simulink model "simulation32"  (R2015b)
settings: Solver=VariableStepAuto  StartTime=0.0  StopTime=1500  RelTol=1e-3
values from neighbouring files (symbols this model uses):
  A = [ ... (first row only)    [stateSpaceModel.m]
  B = [ ... (first row only)    [stateSpaceModel.m]
  C = [ ... (first row only)    [stateSpaceModel.m]
  C_2 = [ ... (first row only)    [stateSpaceModel.m]
  D = [ ... (first row only)    [stateSpaceModel.m]
  D_2 = [ ... (first row only)    [stateSpaceModel.m]
  g = 9.81    [constantsForControlGains.m]
  step_course_hold = 25    [stepsForCourseHoldAndManeuvers.m]
  step_course_hold_start_time = 200    [stepsForCourseHoldAndManeuvers.m]
  step_manuever1 = 20    [stepsForCourseHoldAndManeuvers.m]
  step_manuever1_start_time = 200    [stepsForCourseHoldAndManeuvers.m]
  step_manuever2 = 60    [stepsForCourseHoldAndManeuvers.m]
  step_manuever2_start_time = 400    [stepsForCourseHoldAndManeuvers.m]
  step_manuever3 = 70    [stepsForCourseHoldAndManeuvers.m]
  step_manuever3_start_time = 600    [stepsForCourseHoldAndManeuvers.m]
  step_manuever4 = -50    [stepsForCourseHoldAndManeuvers.m]
  step_manuever4_start_time = 800    [stepsForCourseHoldAndManeuvers.m]
  step_manuever5 = -80    [stepsForCourseHoldAndManeuvers.m]
  step_manuever5_start_time = 1000    [stepsForCourseHoldAndManeuvers.m]
  step_manuever6 = -60    [stepsForCourseHoldAndManeuvers.m]
  step_manuever6_start_time = 1200    [stepsForCourseHoldAndManeuvers.m]
  T = 20    [stepsForCourseHoldAndManeuvers.m]
  Va = 552/3.6    (= 153.333333333)    [constantsForControlGains.m]
undefined symbols (not defined in the file or in its folder): Kp, Kphi, Kr, T_chi, Tw
libraries: simulink_extras x11
settings Model: Creator=ShivJeet  LastModifiedBy=ShivJeet

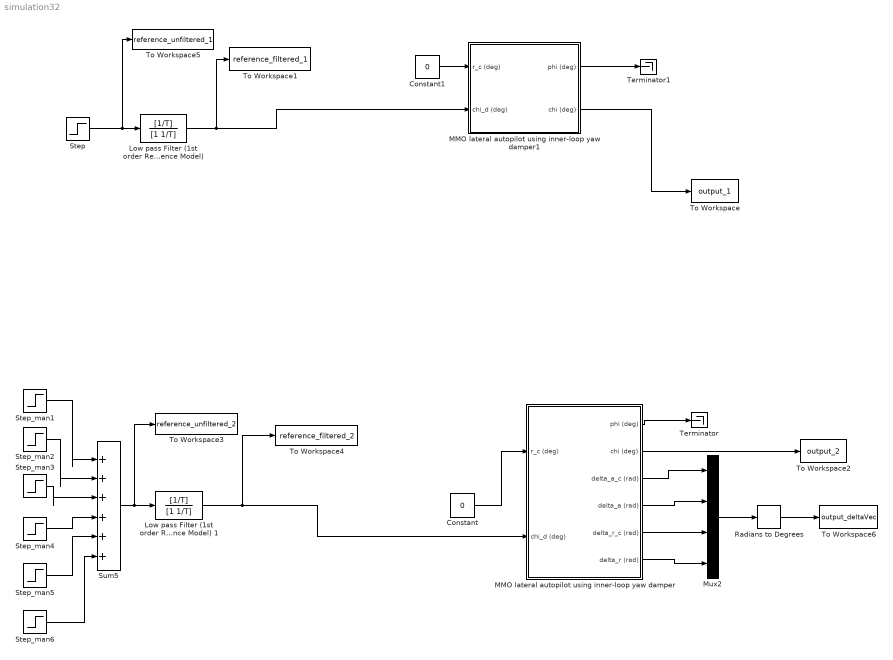
== system simulation32 ==
  Constant : Constant  Value=0
  Constant1 : Constant  Value=0
  "Low pass Filter (1st order Reference Model) " : TransferFcn  Numerator=[1/T]  Denominator=[1 1/T]
  Low pass Filter (1st order Reference Model) 1 : TransferFcn  Numerator=[1/T]  Denominator=[1 1/T]
  MMO lateral autopilot using inner-loop yaw damper : Subsystem
  MMO lateral autopilot using inner-loop yaw damper1 : Subsystem
  Mux2 : Mux
  Radians to Degrees : simulink_extras/Transformations/Radians to Degrees
  Step : Step  Time=step_course_hold_start_time  After=step_course_hold  SampleTime=0
  Step_man1 : Step  Time=step_manuever1_start_time  After=step_manuever1  SampleTime=0
  Step_man2 : Step  Time=step_manuever2_start_time  After=step_manuever2  SampleTime=0
  Step_man3 : Step  Time=step_manuever3_start_time  After=step_manuever3  SampleTime=0
  Step_man4 : Step  Time=step_manuever4_start_time  After=step_manuever4  SampleTime=0
  Step_man5 : Step  Time=step_manuever5_start_time  After=step_manuever5  SampleTime=0
  Step_man6 : Step  Time=step_manuever6_start_time  After=step_manuever6  SampleTime=0
  Sum5 : Sum  Inputs=|++++++
  Terminator : Terminator
  Terminator1 : Terminator
  To Workspace : ToWorkspace  VariableName=output_1  SaveFormat=Timeseries  SampleTime=-1
  To Workspace1 : ToWorkspace  VariableName=reference_filtered_1  SaveFormat=Timeseries  SampleTime=-1
  To Workspace2 : ToWorkspace  VariableName=output_2  SaveFormat=Timeseries  SampleTime=-1
  To Workspace3 : ToWorkspace  VariableName=reference_unfiltered_2  SaveFormat=Timeseries  SampleTime=-1
  To Workspace4 : ToWorkspace  VariableName=reference_filtered_2  SaveFormat=Timeseries  SampleTime=-1
  To Workspace5 : ToWorkspace  VariableName=reference_unfiltered_1  SaveFormat=Timeseries  SampleTime=-1
  To Workspace6 : ToWorkspace  VariableName=output_deltaVec  SaveFormat=Timeseries  SampleTime=-1
  wires:
  MMO lateral autopilot using inner-loop yaw damper/1(phi (deg)) -> Terminator/1
  Constant/1 -> MMO lateral autopilot using inner-loop yaw damper/1(r_c (deg))
  Constant1/1 -> MMO lateral autopilot using inner-loop yaw damper1/1(r_c (deg))
  MMO lateral autopilot using inner-loop yaw damper1/1(phi (deg)) -> Terminator1/1
  MMO lateral autopilot using inner-loop yaw damper/3(delta_a_c (rad)) -> Mux2/1
  MMO lateral autopilot using inner-loop yaw damper/4(delta_a (rad)) -> Mux2/2
  MMO lateral autopilot using inner-loop yaw damper/5(delta_r_c (rad)) -> Mux2/3
  MMO lateral autopilot using inner-loop yaw damper/6(delta_r (rad)) -> Mux2/4
  Mux2/1 -> Radians to Degrees/1
  Radians to Degrees/1 -> To Workspace6/1
  Sum5/1 -> To Workspace3/1, Low pass Filter (1st order Reference Model) 1/1
  Step_man1/1 -> Sum5/1
  Step_man2/1 -> Sum5/2
  Step_man3/1 -> Sum5/3
  Step_man4/1 -> Sum5/4
  Step_man5/1 -> Sum5/5
  Step_man6/1 -> Sum5/6
  Low pass Filter (1st order Reference Model) 1/1 -> MMO lateral autopilot using inner-loop yaw damper/2(chi_d (deg)), To Workspace4/1
  Step/1 -> To Workspace5/1, "Low pass Filter (1st order Reference Model) "/1
  "Low pass Filter (1st order Reference Model) "/1 -> MMO lateral autopilot using inner-loop yaw damper1/2(chi_d (deg)), To Workspace1/1
  MMO lateral autopilot using inner-loop yaw damper/2(chi (deg)) -> To Workspace2/1
  MMO lateral autopilot using inner-loop yaw damper1/2(chi (deg)) -> To Workspace/1

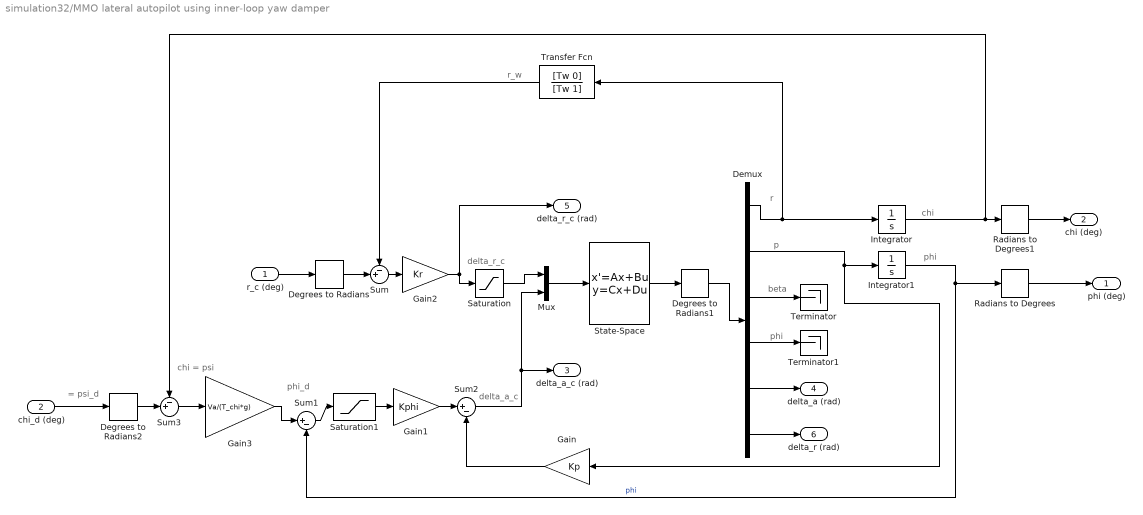
== system simulation32/MMO lateral autopilot using inner-loop yaw damper ==
  note: phi
  note: delta_a_c
  note: chi = psi
  note: = psi_d
  note: phi_d
  note: delta_r_c
  note: r_w
  note: phi
  note: chi
  note: beta
  note: p
  note: r
  r_c (deg) : Inport
  chi_d (deg) : Inport  Port=2
  Degrees to Radians : simulink_extras/Transformations/Degrees to Radians
  Degrees to Radians1 : simulink_extras/Transformations/Degrees to Radians
  Degrees to Radians2 : simulink_extras/Transformations/Degrees to Radians
  Demux : Demux  Outputs=6
  Gain : Gain  Gain=Kp
  Gain1 : Gain  Gain=Kphi
  Gain2 : Gain  Gain=Kr
  Gain3 : Gain  Gain=Va/(T_chi*g)
  Integrator : Integrator
  Integrator1 : Integrator
  Mux : Mux  Inputs=2
  Radians to Degrees : simulink_extras/Transformations/Radians to Degrees
  Radians to Degrees1 : simulink_extras/Transformations/Radians to Degrees
  Saturation : Saturate  UpperLimit=45 * pi/180  LowerLimit=- 45 * pi/180
  Saturation1 : Saturate  UpperLimit=15 * pi/180  LowerLimit=- 15 * pi/180
  State-Space : StateSpace  A=A  B=B  C=C_2  D=D_2  X0=0
  Sum : Sum  Inputs=-+|
  Sum1 : Sum  Inputs=|+-
  Sum2 : Sum  Inputs=|+-
  Sum3 : Sum  Inputs=-+|
  Terminator : Terminator
  Terminator1 : Terminator
  Transfer Fcn : TransferFcn  Numerator=[Tw 0]  Denominator=[Tw 1]
  phi (deg) : Outport
  chi (deg) : Outport  Port=2
  delta_a_c (rad) : Outport  Port=3
  delta_a (rad) : Outport  Port=4
  delta_r_c (rad) : Outport  Port=5
  delta_r (rad) : Outport  Port=6
  wires:
  Integrator1/1 -> Radians to Degrees/1, Sum1/2  "phi"
  Demux/3 -> Terminator/1
  Sum2/1 -> delta_a_c (rad)/1, Mux/2
  Demux/1 -> Transfer Fcn/1, Integrator/1
  Demux/2 -> Gain/1, Integrator1/1
  Sum/1 -> Gain2/1
  State-Space/1 -> Degrees to Radians1/1
  r_c (deg)/1 -> Degrees to Radians/1
  Integrator/1 -> Sum3/1, Radians to Degrees1/1
  Transfer Fcn/1 -> Sum/1
  Degrees to Radians2/1 -> Sum3/2
  Degrees to Radians/1 -> Sum/2
  Degrees to Radians1/1 -> Demux/1
  Gain3/1 -> Sum1/1
  Radians to Degrees1/1 -> chi (deg)/1
  Radians to Degrees/1 -> phi (deg)/1
  chi_d (deg)/1 -> Degrees to Radians2/1
  Demux/4 -> Terminator1/1
  Sum1/1 -> Saturation1/1
  Gain1/1 -> Sum2/1
  Mux/1 -> State-Space/1
  Sum3/1 -> Gain3/1
  Gain/1 -> Sum2/2
  Demux/5 -> delta_a (rad)/1
  Demux/6 -> delta_r (rad)/1
  Gain2/1 -> delta_r_c (rad)/1, Saturation/1
  Saturation1/1 -> Gain1/1
  Saturation/1 -> Mux/1

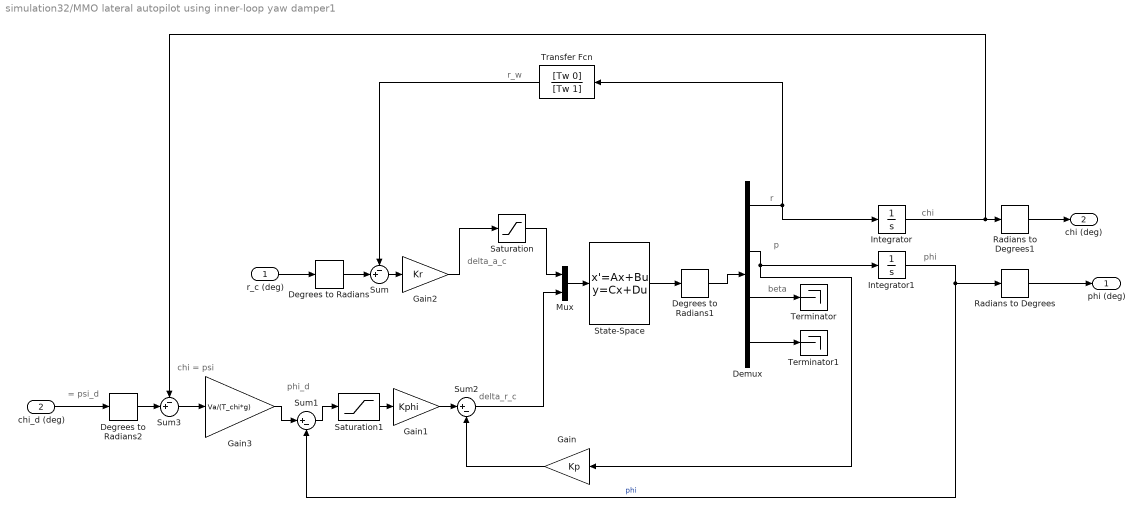
== system simulation32/MMO lateral autopilot using inner-loop yaw damper1 ==
  note: delta_r_c
  note: chi = psi
  note: = psi_d
  note: phi_d
  note: delta_a_c
  note: r_w
  note: phi
  note: chi
  note: beta
  note: p
  note: r
  r_c (deg) : Inport
  chi_d (deg) : Inport  Port=2
  Degrees to Radians : simulink_extras/Transformations/Degrees to Radians
  Degrees to Radians1 : simulink_extras/Transformations/Degrees to Radians
  Degrees to Radians2 : simulink_extras/Transformations/Degrees to Radians
  Demux : Demux
  Gain : Gain  Gain=Kp
  Gain1 : Gain  Gain=Kphi
  Gain2 : Gain  Gain=Kr
  Gain3 : Gain  Gain=Va/(T_chi*g)
  Integrator : Integrator
  Integrator1 : Integrator
  Mux : Mux  Inputs=2
  Radians to Degrees : simulink_extras/Transformations/Radians to Degrees
  Radians to Degrees1 : simulink_extras/Transformations/Radians to Degrees
  Saturation : Saturate  UpperLimit=45 * pi/180  LowerLimit=- 45 * pi/180
  Saturation1 : Saturate  UpperLimit=15 * pi/180  LowerLimit=- 15 * pi/180
  State-Space : StateSpace  A=A  B=B  C=C  D=D  X0=0
  Sum : Sum  Inputs=-+|
  Sum1 : Sum  Inputs=|+-
  Sum2 : Sum  Inputs=|+-
  Sum3 : Sum  Inputs=-+|
  Terminator : Terminator
  Terminator1 : Terminator
  Transfer Fcn : TransferFcn  Numerator=[Tw 0]  Denominator=[Tw 1]
  phi (deg) : Outport
  chi (deg) : Outport  Port=2
  wires:
  Integrator1/1 -> Radians to Degrees/1, Sum1/2  "phi"
  Demux/3 -> Terminator/1
  Sum2/1 -> Mux/2
  Demux/1 -> Transfer Fcn/1, Integrator/1
  Demux/2 -> Gain/1, Integrator1/1
  Sum/1 -> Gain2/1
  State-Space/1 -> Degrees to Radians1/1
  r_c (deg)/1 -> Degrees to Radians/1
  Integrator/1 -> Sum3/1, Radians to Degrees1/1
  Transfer Fcn/1 -> Sum/1
  Degrees to Radians2/1 -> Sum3/2
  Degrees to Radians/1 -> Sum/2
  Degrees to Radians1/1 -> Demux/1
  Gain3/1 -> Sum1/1
  Radians to Degrees1/1 -> chi (deg)/1
  Radians to Degrees/1 -> phi (deg)/1
  chi_d (deg)/1 -> Degrees to Radians2/1
  Demux/4 -> Terminator1/1
  Gain1/1 -> Sum2/1
  Gain2/1 -> Saturation/1
  Mux/1 -> State-Space/1
  Sum3/1 -> Gain3/1
  Gain/1 -> Sum2/2
  Saturation/1 -> Mux/1
  Saturation1/1 -> Gain1/1
  Sum1/1 -> Saturation1/1
